simulink model "num6"  (R2019a)
settings: Solver=VariableStepAuto  StartTime=0.0  StopTime=10.0  RelTol=1e-3
undefined symbols (not defined in the file): C, GZ, HZ, KESCALON, KI, LO
settings Model: Creator=julia  LastModifiedBy=julia

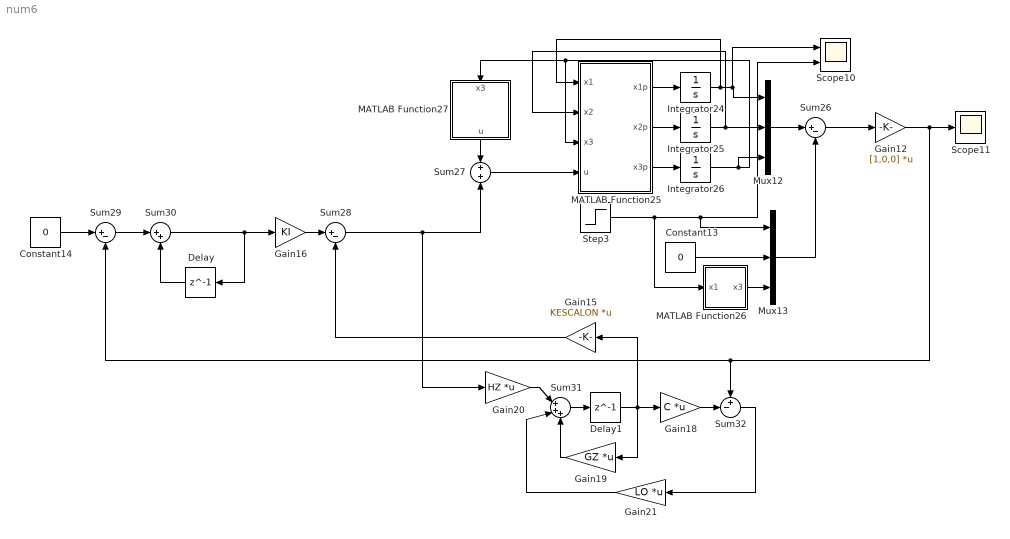
== system num6 ==
  Constant13 : Constant  Value=0
  Constant14 : Constant  Value=0
  Delay : Delay  DelayLength=1  SampleTime=0.05
  Delay1 : Delay  DelayLength=1  SampleTime=0.05
  Gain12 : Gain  Gain=[1,0,0]  Multiplication=Matrix(K*u)
  Gain15 : Gain  Gain=KESCALON  Multiplication=Matrix(K*u)
  Gain16 : Gain  Gain=KI
  Gain18 : Gain  Gain=C  Multiplication=Matrix(K*u)
  Gain19 : Gain  Gain=GZ  Multiplication=Matrix(K*u)
  Gain20 : Gain  Gain=HZ  Multiplication=Matrix(K*u)
  Gain21 : Gain  Gain=LO  Multiplication=Matrix(K*u)
  Integrator24 : Integrator  InitialCondition=5e-3
  Integrator25 : Integrator
  Integrator26 : Integrator
  MATLAB Function25 : MATLAB Function  TreatAsAtomicUnit=on
  MATLAB Function26 : MATLAB Function  TreatAsAtomicUnit=on
  MATLAB Function27 : MATLAB Function  TreatAsAtomicUnit=on
  Mux12 : Mux  Inputs=3
  Mux13 : Mux  Inputs=3
  Scope10 : Scope  NumInputPorts=2
  Scope11 : Scope
  Step3 : Step  Time=0  Before=5e-3  After=10e-3  SampleTime=0
  Sum26 : Sum  Inputs=|+-
  Sum27 : Sum  Inputs=+|+
  Sum28 : Sum  Inputs=|+-
  Sum29 : Sum  Inputs=|+-
  Sum30 : Sum  Inputs=|++
  Sum31 : Sum  Inputs=|+++
  Sum32 : Sum  Inputs=+-|
  wires:
  Sum26/1 -> Gain12/1
  Gain15/1 -> Sum28/2
  Constant14/1 -> Sum29/1
  Gain12/1 -> Sum29/2, Sum32/1, Scope11/1
  Gain16/1 -> Sum28/1
  MATLAB Function27/1(u) -> Sum27/1
  Sum27/1 -> MATLAB Function25/4(u)
  Mux13/1 -> Sum26/2
  MATLAB Function26/1(x3) -> Mux13/3
  Step3/1 -> Mux13/1, Scope10/2, MATLAB Function26/1(x1)
  Constant13/1 -> Mux13/2
  Mux12/1 -> Sum26/1
  Integrator26/1 -> Mux12/3, MATLAB Function25/3(x3), MATLAB Function27/1(x3)
  Integrator25/1 -> Mux12/2, MATLAB Function25/2(x2)
  Integrator24/1 -> Mux12/1, Scope10/1, MATLAB Function25/1(x1)
  MATLAB Function25/3(x3p) -> Integrator26/1
  MATLAB Function25/2(x2p) -> Integrator25/1
  MATLAB Function25/1(x1p) -> Integrator24/1
  Sum30/1 -> Gain16/1, Delay/1
  Delay/1 -> Sum30/2
  Sum29/1 -> Sum30/1
  Sum32/1 -> Gain21/1
  Delay1/1 -> Gain19/1, Gain18/1, Gain15/1
  Gain19/1 -> Sum31/3
  Sum31/1 -> Delay1/1
  Gain18/1 -> Sum32/2
  Gain20/1 -> Sum31/1
  Gain21/1 -> Sum31/2
  Sum28/1 -> Sum27/2, Gain20/1

== matlab function num6/MATLAB Function25 ==
  data: x1 input size=1; x1p output size=1; x2 input size=1; x3 input size=1; x2p output size=1; x3p output size=1; u input size=1
function [x1p,x2p,x3p] = planta(x1,x2,x3,u)
c=0.1;
m=0.01;
L=100e-3;
r=10;
g=9.81;

x1p=x2;
x2p=g-(c/m)*((x3^2)/x1);
x3p=-(r/L)*x3+(1/L)*u;

== matlab function num6/MATLAB Function26 ==
  data: x1 input size=1; x3 output size=1
function x3  = fcn(x1)
c=1
m=0.1
L=0.01
r=1
g=9.81

x3=sqrt((m*g*x1)/c);

== matlab function num6/MATLAB Function27 ==
  data: x3 input size=1; u output size=1
function u  = u(x3)
c=1
m=0.1
L=0.01
r=1
g=9.81

u=r*x3;
